simulink model "ampl_modul"  (R2024a)
settings: Solver=VariableStepAuto  StartTime=0.0  StopTime=16.0  MaxStep=0.01  RelTol=1e-3
settings Model: Creator=DNS  LastModifiedBy=DNS

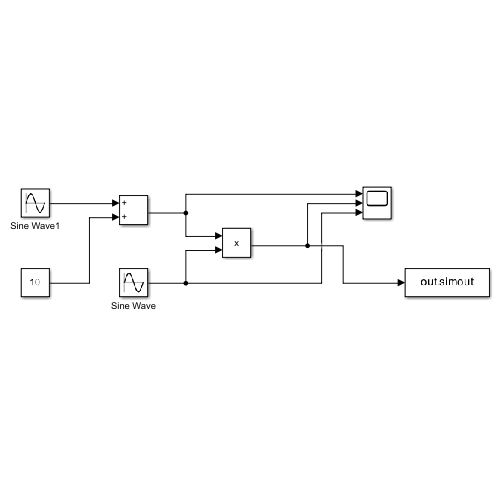
[thumbnail: Simulink's stored preview of the top-level diagram]
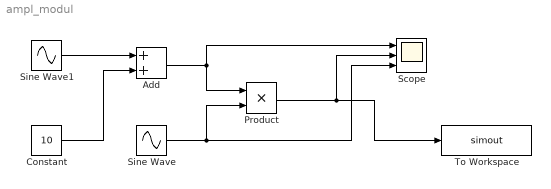
== system ampl_modul ==
  Add : Sum
  Constant : Constant  Value=10
  Product : Product
  Scope : Scope  NumInputPorts=3
  Sine Wave : Sin  Frequency=2*pi*5  SampleTime=0
  Sine Wave1 : Sin  Amplitude=10*5/15  Frequency=2*pi*0.1  SampleTime=0
  To Workspace : ToWorkspace  VariableName=simout  SaveFormat=Structure With Time  SampleTime=-1
  wires:
  Sine Wave1/1 -> Add/1
  Constant/1 -> Add/2
  Add/1 -> Scope/1, Product/1
  Sine Wave/1 -> Scope/3, Product/2
  Product/1 -> To Workspace/1, Scope/2
